simulink model "Task3_FloorSignal"  (R2025a)
settings: Solver=FixedStepDiscrete  StartTime=0.0  StopTime=40  FixedStep=1e-5  RelTol=1e-3
model workspace (MAT data in the model file):
  d = Simulink.Parameter
  d.Value = 0.005
  d.Complexity = 'real'
  d.Dimensions = [1 1]
  d.DataType = 'auto'
  v = Simulink.Parameter
  v.Value = 3
  v.Complexity = 'real'
  v.Dimensions = [1 1]
  v.DataType = 'auto'
  w = Simulink.Parameter
  w.Value = 0.01
  w.Complexity = 'real'
  w.Dimensions = [1 1]
  w.DataType = 'auto'
libraries: simulink x2
settings Model: Creator=randi  LastModifiedBy=randi

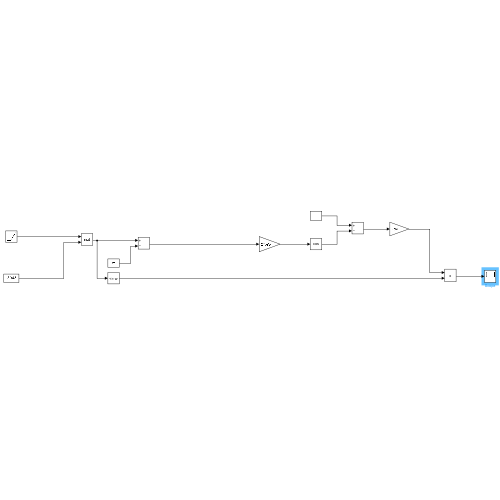
[thumbnail: Simulink's stored preview of the top-level diagram]
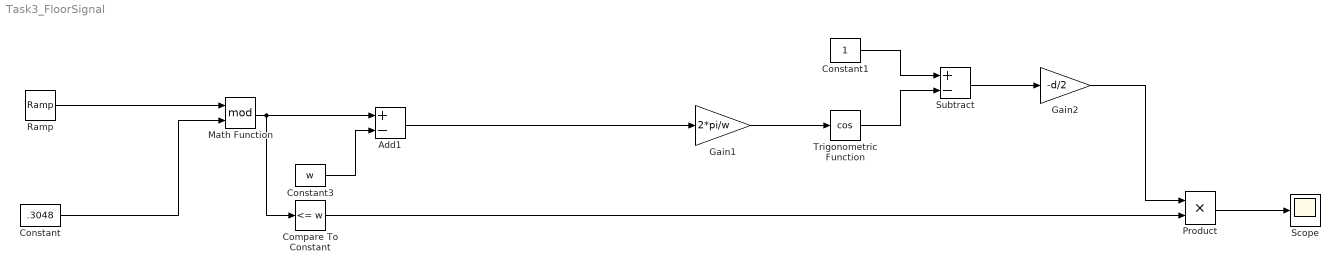
== system Task3_FloorSignal ==
  Add1 : Sum  Inputs=+-
  Compare To Constant : simulink/Logic and Bit Operations/Compare To Constant  relop=<=  const=w  OutDataTypeStr=boolean
  Constant : Constant  Value=.3048
  Constant1 : Constant
  Constant3 : Constant  Value=w
  Gain1 : Gain  Gain=2*pi/w
  Gain2 : Gain  Gain=-d/2
  Math Function : Math  Operator=mod
  Product : Product
  Ramp : simulink/Sources/Ramp  slope=v  start=0  InitialOutput=0
  Scope : Scope
      settings: ActiveDisplayYMinimum=-0.0050654392073922559  ActiveDisplayYMaximum=6.1859948097581785E-5
  Subtract : Sum  Inputs=+-
  Trigonometric Function : Trigonometry  Operator=cos
  wires:
  Gain1/1 -> Trigonometric Function/1
  Trigonometric Function/1 -> Subtract/2
  Constant1/1 -> Subtract/1
  Subtract/1 -> Gain2/1
  Constant/1 -> Math Function/2
  Ramp/1 -> Math Function/1
  Constant3/1 -> Add1/2
  Add1/1 -> Gain1/1
  Math Function/1 -> Compare To Constant/1, Add1/1
  Gain2/1 -> Product/1
  Compare To Constant/1 -> Product/2
  Product/1 -> Scope/1
